simulink model "bicycle_model"  (R2025a)
settings: Solver=VariableStepAuto  StartTime=0.0  StopTime=5  MaxStep=0.001  RelTol=1e-3
undefined symbols (not defined in the file): a, A, b, B, beta_th, C, Cf, Cr, D, er_th, Fbrk_max, Fy_f_max, Fy_r_max, Iz, Kbeta, Kr, L, lambda_off, lambda_on, m, Mz_max, r_fric, tau, tau_ay, track, Ux
libraries: simulink x4
settings Model: NumberOfSteps=2  Creator=muhan  LastModifiedBy=muhan
settings SolverCC: ZeroCrossAlgorithm=Adaptive
settings DebuggingCC: IgnoredZcDiagnostic=none

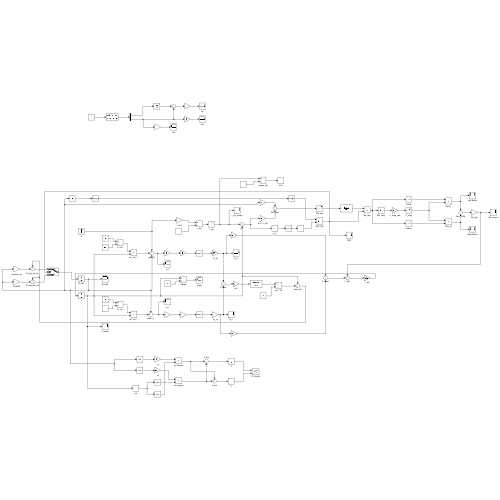
[thumbnail: Simulink's stored preview of the top-level diagram]
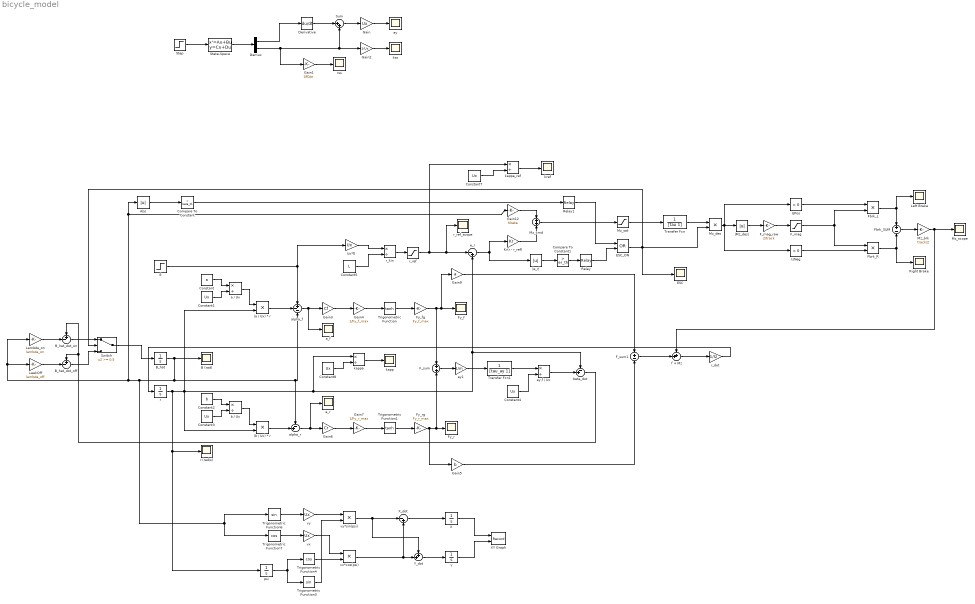
== system bicycle_model ==
  (a / Ux) * r : Product
  (b / Ux) * r : Product
  Abs : Abs  SaturateOnIntegerOverflow=off
  B (rad) : Scope
      settings: ActiveDisplayYMinimum=-0.86910030568136254  ActiveDisplayYMaximum=0.10009196576314162  DataLoggingVariableName=ScopeData10
  B_hat : Integrator
  B_hat_dot_off : Sum  Inputs=+-|
  "B_hat_dot_on " : Sum  Inputs=+-|
  Compare To Constant : simulink/Logic and Bit Operations/Compare To Constant  relop=>  const=beta_th  OutDataTypeStr=boolean  ZeroCross=off
  Compare To Constant1 : simulink/Logic and Bit Operations/Compare To Constant  relop=>  const=er_th  OutDataTypeStr=boolean  ZeroCross=off
  Constant : Constant  Value=a
  Constant{1,3..4,7..8} (5 alike) : Constant  Value=Ux
  Constant2 : Constant  Value=b
  Constant5 : Constant  Value=L
  Demux : Demux  Outputs=2
  Derivative : Derivative
  ESC : Scope
      settings: ActiveDisplayYMinimum=-0.12499999999999997  ActiveDisplayYMaximum=1.125  DataLoggingVariableName=ScopeData11
  ESC_ON : Logic  Operator=OR  AllPortsSameDT=off  OutDataTypeStr=boolean
  F_mag : Saturate  UpperLimit=Fbrk_max  LowerLimit=0
  F_mag_raw : Gain  Gain=2/track
  F_sum : Sum
  F_sum1 : Sum  Inputs=+-
  Fbrk_L : Product
  Fbrk_R : Product
  Fbrk_SUM : Sum  Inputs=+-
  Fy_f : Scope
      settings: ActiveDisplayYMinimum=5460.5440620069958  ActiveDisplayYMaximum=16426.364309320743  DataLoggingVariableName=ScopeData3
  Fy_fg : Gain  Gain=Fy_f_max
  Fy_r : Scope
      settings: ActiveDisplayYMinimum=-7447.4999999997535  ActiveDisplayYMaximum=827.49999999997237  DataLoggingVariableName=ScopeData4
  Fy_rg : Gain  Gain=Fy_r_max
  Gain : Gain  Gain=Ux
  Gain1 : Gain  Gain=180/pi
  Gain12 : Gain  Gain=Kbeta
  Gain2 : Gain  Gain=1/Ux
  Gain3 : Gain  Gain=Cf
  Gain4 : Gain  Gain=1/Fy_f_max
  Gain5 : Gain  Gain=b
  Gain6 : Gain  Gain=Cr
  Gain7 : Gain  Gain=1/Fy_r_max
  Gain9 : Gain  Gain=a
  IsNeg : simulink/Logic and Bit Operations/Compare To Zero  relop=<  OutDataTypeStr=boolean
  IsPos : simulink/Logic and Bit Operations/Compare To Zero  relop=>  OutDataTypeStr=boolean
  Kr(r - r_ref) : Gain  Gain=Kr
  Lambda_on : Gain  Gain=lambda_on
  LeakOff : Gain  Gain=lambda_off
  Left Brake : Scope
      settings: ActiveDisplayYMinimum=-434.03149204865986  ActiveDisplayYMaximum=3906.2834284379396  DataLoggingVariableName=ScopeData8
  Mz_brk : Gain  Gain=track/2
  Mz_cmd : Sum
  Mz_des : Product
  Mz_sat : Saturate  UpperLimit=Mz_max  LowerLimit=- Mz_max
  Mz_scope : Scope
      settings: ActiveDisplayYMinimum=-1725.2693218311676  ActiveDisplayYMaximum=302.26878401950364  DataLoggingVariableName=ScopeData18
  Relay : Relay  OnSwitchValue=0.15  OffSwitchValue=0.08
  Relay1 : Relay  OnSwitchValue=0.15  OffSwitchValue=0.08
  Right Brake : Scope
      settings: ActiveDisplayYMinimum=-468.29138855766564  ActiveDisplayYMaximum=4214.6224970189915  DataLoggingVariableName=ScopeData14
  State-Space : StateSpace  A=A  B=B  C=C  D=D  InitialCondition=0
  Step : Step  Time=0  After=2*pi/180  SampleTime=0
  Sum : Sum  Inputs=|++
  Switch : Switch  Threshold=0.5  SaturateOnIntegerOverflow=off  InputSameDT=off
  Transfer Fcn : TransferFcn  Denominator=[tau 1]
  Transfer Fcn1 : TransferFcn  Denominator=[tau_ay 1]
  Trigonometric Function : Trigonometry  Operator=tanh
  Trigonometric Function1 : Trigonometry  Operator=tanh
  Trigonometric Function3 : Trigonometry
  Trigonometric Function4 : Trigonometry  Operator=cos
  Trigonometric Function6 : Trigonometry
  Trigonometric Function7 : Trigonometry  Operator=cos
  Ux*δ : Gain  Gain=Ux
  X : Integrator
  XY Graph : Record  NumPorts=2.0  FileSettingsInternal="{\"entries\":[{\"content\":{\"excelSettings\":{\"content\":{},\"type\":\"Streamout.ExcelSettings\"},\"parquetSettings\":{\"content\":{},\"type\":\"Streamout.ParquetSettings\"}},\"type\":\"Streamout.FileSettingStorage\",\"uuid\":\"\"}],\"packageUris\":[\"http:\\/\\/schema.mathworks.com\\/mf0\\/streamout_blocks\\/R2020a\"],\"version\":\"1.0\"}"  FrameSettings=[0, 0]  Layout=[1 1]  SignalsInternal="{\"entries\":[{\"content\":{\"signals\":[{\"content\":{\"blockPath\":[],\"dimensions\":[1],\"domain\":\"\",\"lineColor\":\"#a2142f\",\"plots\":[ 1 ],\"port\":1,\"sid\":[\"\"],\"signalID\":1,\"signalName\":\"X\"},\"type\":\"RecordBlkView.Signal\",\"uuid\":\"\"},{\"content\":{\"blockPath\":[],\"dimensions\":[1],\"domain\":\"\",\"lineColor\":\"#139fff\",\"plots\":[ 1 ],\"port\":2,\"sid\":[\"\"],\"signalID\":2,\"signalName\":\"Y\"},\"type\":\"RecordBlkView.Signal\",\"uuid\":\"\"}]},\"type\":\"RecordBlkView.InputSignals\",\"uuid\":\"\"}],\"packageUris\":[\"http:\\/\\/schema.mathworks.com\\/mf0\\/streamout_blocks\\/R2020a\"],\"version\":\"1.0\"}"  VisualizationBindings="{\"xyplotplugin\":{\"info\":[{\"series\":[{\"bindingParametersList\":[{\"parameter\":\"X-Axis\",\"signalID\":1,\"signalName\":\"X\"},{\"parameter\":\"Y-Axis\",\"signalID\":2,\"signalName\":\"Y\"},{\"parameter\":\"X-Axis\",\"signalID\":1,\"signalName\":\"X\"},{\"parameter\":\"Y-Axis\",\"signalID\":2,\"signalName\":\"Y\"},{\"parameter\":\"X-Axis\",\"signalID\":1,\"signalName\":\"X\"},{\"parameter\":\"Y-Axis\",\"signalID\":2,\"signalName\":\"Y\"}],\"seriesID\":0}],\"subplotID\":1}]}}"  CompatibilityTag=XY
  X_dot : Sum  Inputs=|-+
  Y : Integrator
  Y_dot : Sum  Inputs=++|
  a / Ux : Product  Inputs=*/
  a_f : Scope
      settings: ActiveDisplayYMinimum=0.08601888353846722  ActiveDisplayYMaximum=0.62209344974925873  DataLoggingVariableName=ScopeData5
  a_r : Scope
      settings: ActiveDisplayYMinimum=-0.053607456621079137  ActiveDisplayYMaximum=0.48246710958971234  DataLoggingVariableName=ScopeData6
  alpha_f : Sum  Inputs=+--
  alpha_r : Sum  Inputs=-+|
  ay : Scope
      settings: ActiveDisplayYMinimum=-9.5654915450519589  ActiveDisplayYMaximum=9.72895135835865
  ay,f / Ux : Product  Inputs=*/
  ay1 : Gain  Gain=1/m
  b / Ux : Product  Inputs=*/
  beta_dot : Sum  Inputs=-+|
  e_r : Sum  Inputs=|-+
  f + Mz : Sum  Inputs=++|
  kapp : Scope
      settings: ActiveDisplayYMinimum=-0.0041607643217965494  ActiveDisplayYMaximum=0.037446878896168954  DataLoggingVariableName=ScopeData7
  kappa : Product  Inputs=*/
  kappa_ref : Product  Inputs=*/
  kref : Scope
      settings: ActiveDisplayYMinimum=-0.032072500000000004  ActiveDisplayYMaximum=-0.012072500000000002  DataLoggingVariableName=ScopeData9
  kss : Scope
      settings: ActiveDisplayYMinimum=-0.033107291847622476  ActiveDisplayYMaximum=0.048594343159297  DataLoggingVariableName=ScopeData2
  psi : Integrator
  r : Integrator
  r (rad/s) : Scope
      settings: ActiveDisplayYMinimum=-0.083215286435931  ActiveDisplayYMaximum=0.74893757792337912  DataLoggingVariableName=ScopeData13
  r_dot : Gain  Gain=1/Iz
  r_kin : Product  Inputs=*/
  r_ref : Saturate  UpperLimit=r_fric  LowerLimit=- r_fric
  r_ref_scope : Scope
      settings: ActiveDisplayYMinimum=0.34145000000000003  ActiveDisplayYMaximum=0.54145  DataLoggingVariableName=ScopeData15
  rss : Scope
      settings: ActiveDisplayYMinimum=-8.3829563783730769  ActiveDisplayYMaximum=13.63504359290544
  vx : Gain  Gain=Ux
  vx*cos(psi) : Product
  vy : Gain  Gain=Ux
  vy*sin(psi) : Product
  |Mz_des| : Abs  SaturateOnIntegerOverflow=off
  |e_r| : Abs  SaturateOnIntegerOverflow=off
  δ : Step  Time=0  After=8*pi/180  SampleTime=0
  wires:
  Step/1 -> State-Space/1
  State-Space/1 -> Demux/1
  Demux/2 -> Gain2/1, Sum/2, Gain1/1
  Gain1/1 -> rss/1
  Gain/1 -> ay/1
  Demux/1 -> Derivative/1
  Derivative/1 -> Sum/1
  Sum/1 -> Gain/1
  Gain2/1 -> kss/1
  Constant/1 -> a / Ux/1
  Constant1/1 -> a / Ux/2
  a / Ux/1 -> (a / Ux) * r/1
  (a / Ux) * r/1 -> alpha_f/2
  Constant2/1 -> b / Ux/1
  b / Ux/1 -> (b / Ux) * r/1
  (b / Ux) * r/1 -> alpha_r/2
  Constant3/1 -> b / Ux/2
  δ/1 -> Ux*δ/1, alpha_f/1
  alpha_f/1 -> a_f/1, Gain3/1
  Gain3/1 -> Gain4/1
  Gain4/1 -> Trigonometric Function/1
  Trigonometric Function/1 -> Fy_fg/1
  Fy_fg/1 -> Fy_f/1, Gain9/1, F_sum/1
  Trigonometric Function1/1 -> Fy_rg/1
  Gain7/1 -> Trigonometric Function1/1
  Fy_rg/1 -> Gain5/1, F_sum/2, Fy_r/1
  alpha_r/1 -> a_r/1, Gain6/1
  Gain6/1 -> Gain7/1
  F_sum/1 -> ay1/1
  Constant4/1 -> ay,f / Ux/2
  ay,f / Ux/1 -> beta_dot/2
  beta_dot/1 -> "B_hat_dot_on "/1, B_hat_dot_off/1
  Gain9/1 -> F_sum1/1
  Gain5/1 -> F_sum1/2
  r_dot/1 -> r/1
  r/1 -> (a / Ux) * r/2, kappa/1, beta_dot/1, e_r/2, (b / Ux) * r/2, psi/1, r (rad/s)/1
  Ux*δ/1 -> r_kin/1
  Constant5/1 -> r_kin/2
  r_kin/1 -> r_ref/1
  e_r/1 -> Kr(r - r_ref)/1, |e_r|/1
  Gain12/1 -> Mz_cmd/1
  Kr(r - r_ref)/1 -> Mz_cmd/2
  Abs/1 -> Compare To Constant/1
  |e_r|/1 -> Compare To Constant1/1
  Compare To Constant1/1 -> Relay/1
  Compare To Constant/1 -> Relay1/1
  Mz_sat/1 -> Transfer Fcn/1
  ESC_ON/1 -> Switch/2, Mz_des/2, ESC/1
  F_sum1/1 -> f + Mz/2
  f + Mz/1 -> r_dot/1
  Transfer Fcn/1 -> Mz_des/1
  Constant7/1 -> kappa_ref/2
  kappa_ref/1 -> kref/1
  Constant8/1 -> kappa/2
  kappa/1 -> kapp/1
  r_ref/1 -> e_r/1, r_ref_scope/1, kappa_ref/1
  Mz_brk/1 -> Mz_scope/1, f + Mz/1
  Mz_des/1 -> IsPos/1, IsNeg/1, |Mz_des|/1
  |Mz_des|/1 -> F_mag_raw/1
  F_mag_raw/1 -> F_mag/1
  Fbrk_L/1 -> Left Brake/1, Fbrk_SUM/1
  Fbrk_R/1 -> Right Brake/1, Fbrk_SUM/2
  Fbrk_SUM/1 -> Mz_brk/1
  F_mag/1 -> Fbrk_R/1, Fbrk_L/2
  IsPos/1 -> Fbrk_L/1
  IsNeg/1 -> Fbrk_R/2
  Mz_cmd/1 -> Mz_sat/1
  ay1/1 -> Transfer Fcn1/1
  Transfer Fcn1/1 -> ay,f / Ux/1
  LeakOff/1 -> B_hat_dot_off/2
  B_hat_dot_off/1 -> Switch/3
  Switch/1 -> B_hat/1
  Lambda_on/1 -> "B_hat_dot_on "/2
  "B_hat_dot_on "/1 -> Switch/1
  Relay/1 -> ESC_ON/2
  Relay1/1 -> ESC_ON/1
  B_hat/1 -> B (rad)/1, alpha_f/3, alpha_r/1, Trigonometric Function7/1, Trigonometric Function6/1, Lambda_on/1, LeakOff/1, Abs/1, Gain12/1
  Trigonometric Function7/1 -> vx/1
  Trigonometric Function6/1 -> vy/1
  psi/1 -> Trigonometric Function4/1, Trigonometric Function3/1
  vx/1 -> vx*cos(psi)/1
  Trigonometric Function4/1 -> vx*cos(psi)/2
  Trigonometric Function3/1 -> vy*sin(psi)/2
  vy/1 -> vy*sin(psi)/1
  vy*sin(psi)/1 -> X_dot/1, Y_dot/1
  vx*cos(psi)/1 -> Y_dot/2, X_dot/2
  X_dot/1 -> X/1
  Y_dot/1 -> Y/1
  X/1 -> XY Graph/1
  Y/1 -> XY Graph/2
